simulink model "Controller"  (R2026a)
settings: Solver=FixedStepAuto  StopTime=inf  FixedStep=ControllerStepSize  MaxStep=Ts
PreLoadFcn:
  | % Position and velocity selectors from track state
  | % The filter initialization function used in this example is initcvekf that
  | % defines a state that is: [x;vx;y;vy;z;vz].
  | trackPosSelector = [1,0,0,0,0,0; 0,0,1,0,0,0];
  | assignin('base','trackPosSelector',trackPosSelector);
  | 
  | % Width of the ego path for MIO consideration(m)
  | assignin('base','egoPathWidth', single(3.5));
  | 
  | 
  | egoVehDyn.Mass = 1575;
  | egoVehDyn.CGToFrontAxle = 1.5149;
  | egoVehDyn.CGToRearAxle = 1.3042;
  | egoVehDyn.Cf = 19000;
  | assignin('base','egoVehDyn', egoVehDyn);
  | 
  | 
  | maxSteer = 1.13; % Maximum steering angle (rad)
  | assignin('base', 'maxSteer', maxSteer);
undefined symbols (not defined in the file or in its folder): accGapGain, accKi, accKp, accLaneWidth, accMaxAcceleration, accMinAcceleration, accStandstillGap, accTimeHeadway, AEB, ControllerStepSize, egoPathWidth, FCW, LaneWidth, Left, maxDecel, predictionHorizon, Right, Ts
libraries: simulink_extras x8, simulink x2, drivingvehiclecontroller x2, slpidlib x1, mpcadaslib x1
CloseFcn:
  | evalin('base','clear(''trackPosSelector'')');
  | evalin('base','clear(''egoPathWidth'')');
settings Model: Creator=The MathWorks, Inc.  LastModifiedBy=mraj
settings SolverCC: MinimalZcImpactIntegration=on
settings OptimizationCC: InlineInvariantSignals=on  InitFltsAndDblsToZero=on
settings HardwareCC: TargetLongLongMode=on
settings SFSimCC: SimTargetLang=C++
settings RTWCC: SystemTargetFile=ert.tlc  GenerateReport=on  BuildConfiguration=Faster Runs  IncludeHyperlinkInReport=on  LaunchReport=on  TargetLang=C++  GenerateTraceInfo=on  GenerateTraceReport=on  GenerateTraceReportSl=on  GenerateTraceReportSf=on  GenerateTraceReportEml=on  GenerateCodeMetricsReport=on  LargeConstantGeneration=WriteOnlyDNNConstantsToDataFiles  Description=Embedded Coder
settings CodeAppCC: MaxIdLength=63.0  CustomSymbolStrFcn=$N$M$F
settings ERTTargetCC: RootIOFormat=Structure reference  RTWCAPISignals=on  DynamicArrayContainerType=coder::array  TargetLangStandard=C++03 (ISO)  GenerateSampleERTMain=on  CombineSignalStateStructs=on  SuppressErrorStatus=on  CodeInterfacePackaging=C++ class  SupportVariableSizeSignals=on

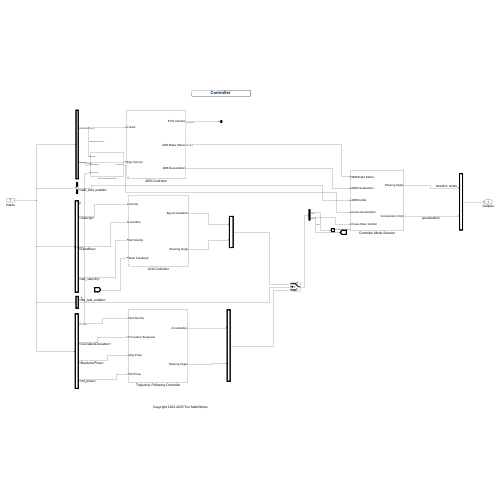
[thumbnail: Simulink's stored preview of the top-level diagram]
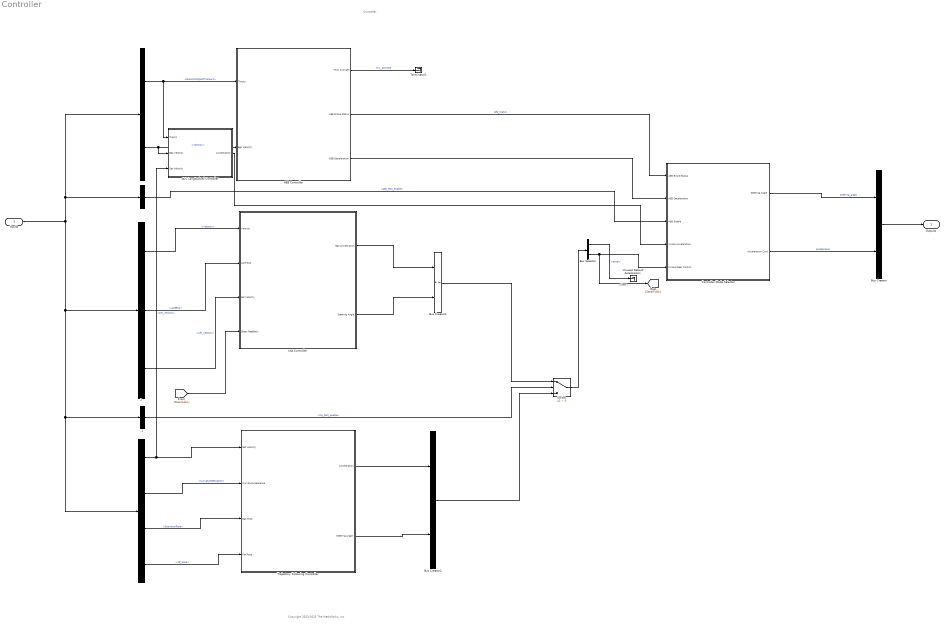
== system Controller ==
  note: Controller
  note: Copyright 2023-2025 The MathWorks, Inc.
  Inputs : Inport  OutDataTypeStr=Bus: BusController  BusOutputAsStruct=on
  "  " : BusSelector  OutputSignals=BusMultiObjectTracker1,BusActorPose.Velocity
  "    " : BusSelector  OutputSignals=set_velocity,BusRefPathInfo.BusDeviations.CurvatureDeviation,BusActorPose,BusRefPathInfo.ref_pose
  "     " : BusSelector  OutputSignals=aeb_test_enable
  "     1" : BusSelector  OutputSignals=lka_test_enable
  "    2" : BusSelector  OutputSignals=BusActorPose.Velocity,LaneBus,set_velocity
  ACC Longitudinal Controller : Subsystem
  AEB Controller : Subsystem  Variant=on  EmptyChoice=on
  Bus Creator : BusCreator  Inputs=2
  Bus Creator1 : BusCreator  Inputs=2  OutDataTypeStr=Bus: AccelSteerBus
      settings: InheritFromInputs=off
  Bus Creator2 : BusCreator  Inputs=2  OutDataTypeStr=Bus: AccelSteerBus
      settings: InheritFromInputs=off
  Bus Selector : BusSelector  OutputSignals=accel,steer
  Controller Mode Selector : Subsystem
  LKA Controller : Subsystem  Variant=on  EmptyChoice=on
  Switch : Switch  Criteria=u2 > Threshold  SaturateOnIntegerOverflow=off  InputSameDT=off  OutDataTypeStr=Inherit: Same as first input
  Terminator1 : Terminator
  Trajectory Following Controller : Subsystem
  Unused Default Acceleration : Terminator
  Outputs : Outport  OutDataTypeStr=Bus: BusVehicleCommands
  wires:
  "     "/1 -> Controller Mode Selector/3(AEB Enable)  "<aeb_test_enable>"
  Bus Creator/1 -> Outputs/1
  "    "/4 -> Trajectory Following Controller/4(Ref Pose)  "<ref_pose>"
  Controller Mode Selector/1(Steering Angle) -> Bus Creator/1  "steering_angle"
  "    "/2 -> Trajectory Following Controller/2(Curvature Sequence)  "<CurvatureDeviation>"
  "    "/3 -> Trajectory Following Controller/3(Ego Pose)  "<BusActorPose>"
  Controller Mode Selector/2(Acceleration Cmd) -> Bus Creator/2  "acceleration"
  Switch/1 -> Bus Selector/1
  Inputs/1 -> "  "/1, "     "/1, "    2"/1, "     1"/1, "    "/1
  "    2"/1 -> LKA Controller/1(Velocity)  "<Velocity>"
  LKA Controller/1(Ego Acceleration) -> Bus Creator1/1
  "    2"/3 -> LKA Controller/3(Set Velocity)  "<set_velocity>"
  "    2"/2 -> LKA Controller/2(Lane Bus)  "<LaneBus>"
  LKA Controller/2(Steering Angle) -> Bus Creator1/2
  Bus Creator1/1 -> Switch/1
  "     1"/1 -> Switch/2  "<lka_test_enable>"
  Bus Creator2/1 -> Switch/3
  Trajectory Following Controller/1(Acceleration) -> Bus Creator2/1
  Trajectory Following Controller/2(Steering Angle) -> Bus Creator2/2
  [SteerFdbk] -> LKA Controller/4(Steer Feedback)
  AEB Controller/1(FCW Activate) -> Terminator1/1  "fcw_activate"
  AEB Controller/2(AEB Brake Status) -> Controller Mode Selector/1(AEB Brake Status)  "aeb_status"
  AEB Controller/3(AEB Deceleration) -> Controller Mode Selector/2(AEB Deceleration)
  Bus Selector/1 -> Unused Default Acceleration/1  "<accel>"
  ACC Longitudinal Controller/1(Acceleration) -> Controller Mode Selector/4(Cruise Acceleration)
  "  "/2 -> ACC Longitudinal Controller/2(Ego Velocity), AEB Controller/2(Ego Velocity)  "<Velocity>"
  "  "/1 -> ACC Longitudinal Controller/1(Tracks), AEB Controller/1(Tracks)  "<BusMultiObjectTracker1>"
  Bus Selector/2 -> [SteerFdbk], Controller Mode Selector/5(Cruise Steer Control)  "<steer>"
  "    "/1 -> ACC Longitudinal Controller/3(Set Velocity), Trajectory Following Controller/1(Set Velocity)  "<set_velocity>"

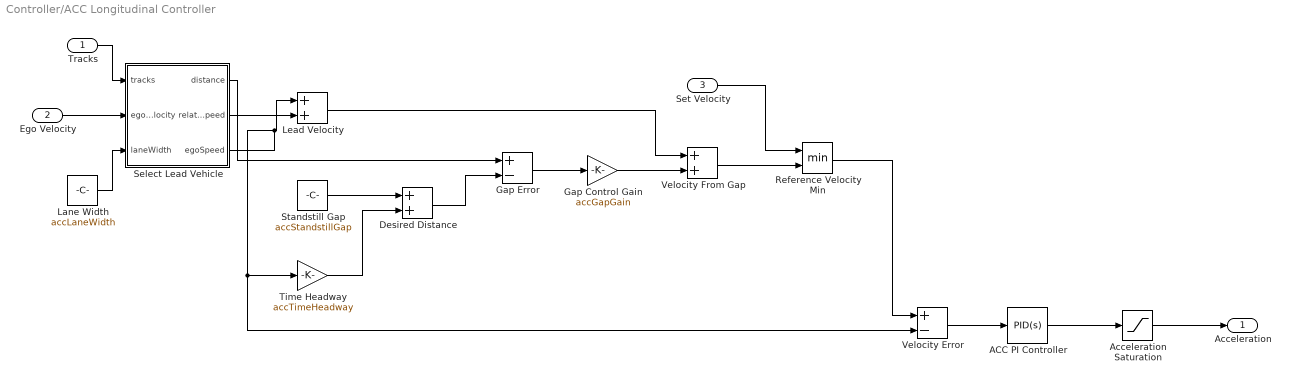
== system Controller/ACC Longitudinal Controller ==
  Tracks : Inport
  Ego Velocity : Inport  Port=2
  Set Velocity : Inport  Port=3
  ACC PI Controller : slpidlib/PID Controller  Controller=PID  Form=Parallel  TimeDomain=Continuous-time  UseExternalTs=off  SampleTime=-1  IntegratorMethod=Forward Euler  FilterMethod=Forward Euler  ControllerParametersSource=internal  P=accKp  I=accKi  UseKiTs=off  D=0  UseExternalDerivativeSource=off  N=100  UseFilter=on  TunerSelectOption=Transfer Function Based (PID Tuner App)  InitialConditionSource=internal  InitialConditionForIntegrator=0  InitialConditionForFilter=0  DifferentiatorICPrevScaledInput=0  ExternalReset=none  TrackingMode=off  Kt=1  LimitOutput=off  SatLimitsSource=internal  UpperSaturationLimit=inf  LowerSaturationLimit=-inf  LinearizeAsGain=on  AntiWindupMode=none  Kb=1  LimitIntegrator=off  UpperIntegratorSaturationLimit=inf  LowerIntegratorSaturationLimit=-inf  POutMin=[]  POutMax=[]  IOutMin=[]  IOutMax=[]  DOutMin=[]  DOutMax=[]  NOutMin=[]  NOutMax=[]  SumOutMin=[]  SumOutMax=[]  SaturationOutMin=[]  SaturationOutMax=[]  PParamMin=[]  PParamMax=[]  IParamMin=[]  IParamMax=[]  DParamMin=[]  DParamMax=[]  NParamMin=[]  NParamMax=[]  KbParamMin=[]  KbParamMax=[]  KtParamMin=[]  KtParamMax=[]  KbOutMin=[]  KbOutMax=[]  KtOutMin=[]  KtOutMax=[]  IntegratorOutMin=[]  IntegratorOutMax=[]  FilterOutMin=[]  FilterOutMax=[]  SumI1OutMin=[]  SumI1OutMax=[]  SumI2OutMin=[]  SumI2OutMax=[]  SumI3OutMin=[]  SumI3OutMax=[]  SumI4OutMin=[]  SumI4OutMax=[]  SumDOutMin=[]  SumDOutMax=[]  DifferentiatorOutMin=[]  DifferentiatorOutMax=[]  FilterDiffOutCoefMin=[]  FilterDiffOutCoefMax=[]  ReciprocalOutMin=[]  ReciprocalOutMax=[]  SumDenOutMin=[]  SumDenOutMax=[]  SumNumOutMin=[]  SumNumOutMax=[]  DivideOutMin=[]  DivideOutMax=[]  UdiffTsProdOutMin=[]  UdiffTsProdOutMax=[]  NTsProdOutMin=[]  NTsProdOutMax=[]  UintegralTsProdOutMin=[]  UintegralTsProdOutMax=[]  UngainTsProdOutMin=[]  UngainTsProdOutMax=[]  ClampingZeroOutDataTypeStr=Inherit: Inherit via back propagation  ClampingZeroOutMin=[]  ClampingZeroOutMax=[]  FilterDenConstantOutDataTypeStr=Inherit: Inherit via back propagation  FilterDenConstantOutMin=[]  FilterDenConstantOutMax=[]  PCopyOutDataTypeStr=Inherit: Inherit via back propagation  PCopyOutMin=[]  PCopyOutMax=[]  NCopyOutDataTypeStr=Inherit: Inherit via back propagation  NCopyOutMin=[]  NCopyOutMax=[]  IntegratorContinuousStateAttributes=''  IntegratorStateMustResolveToSignalObject=off  IntegratorRTWStateStorageClass=Auto  FilterContinuousStateAttributes=''  FilterStateMustResolveToSignalObject=off  FilterRTWStateStorageClass=Auto  ParallelPVariant=InternalParameters  IdealPVariant=Disabled  IVariant=InternalParameters  DVariant=InternalParameters  IntegratorVariant=Continuous  SatVariant=Disabled  AWVariant=Passthrough  PCopyVariant=Disabled  TRVariant=Disabled  FdbkBlocksVariant=Forward  IdealPFdbkVariant=Disabled  SatFdbkVariant=Disabled  DerivativeFilterVariant=ContFilter  NVariant=InternalParameters  NCopyVariant=Disabled  FilterICVariant=InternalICsFilter  IntegratorICVariant=InternalICs  ExternalResetVariant=Disabled  TRSumVariant=Passthrough  SumFdbkVariant=Disabled  SumVariant=Sum_PID  TsampFilterVariant=InternalTs  TsampNgainVariant=Passthrough  TsampIntegralVariant=Disabled_SignalSpec  ExternalSaturationOutDataTypeStr=Inherit: Same as second input  DerivativeSourceVariant=ErrorSignal  PreIntVariant=InternalPreInt
  Acceleration Saturation : Saturate  UpperLimit=accMaxAcceleration  LowerLimit=accMinAcceleration
  Desired Distance : Sum
  Gap Control Gain : Gain  Gain=accGapGain
  Gap Error : Sum  Inputs=+-
  Lane Width : Constant  Value=accLaneWidth
  Lead Velocity : Sum
  Reference Velocity Min : MinMax  Inputs=2
  Select Lead Vehicle : MATLAB Function  TreatAsAtomicUnit=on
  Standstill Gap : Constant  Value=accStandstillGap
  Time Headway : Gain  Gain=accTimeHeadway
  Velocity Error : Sum  Inputs=+-
  Velocity From Gap : Sum
  Acceleration : Outport
  wires:
  Select Lead Vehicle/2(relativeSpeed) -> Lead Velocity/2
  Select Lead Vehicle/3(egoSpeed) -> Time Headway/1, Velocity Error/2, Lead Velocity/1
  Lane Width/1 -> Select Lead Vehicle/3(laneWidth)
  Ego Velocity/1 -> Select Lead Vehicle/2(egoVelocity)
  Tracks/1 -> Select Lead Vehicle/1(tracks)
  Standstill Gap/1 -> Desired Distance/1
  Time Headway/1 -> Desired Distance/2
  Select Lead Vehicle/1(distance) -> Gap Error/1
  Desired Distance/1 -> Gap Error/2
  Gap Error/1 -> Gap Control Gain/1
  Lead Velocity/1 -> Velocity From Gap/1
  Gap Control Gain/1 -> Velocity From Gap/2
  Set Velocity/1 -> Reference Velocity Min/1
  Velocity From Gap/1 -> Reference Velocity Min/2
  Reference Velocity Min/1 -> Velocity Error/1
  Velocity Error/1 -> ACC PI Controller/1
  ACC PI Controller/1 -> Acceleration Saturation/1
  Acceleration Saturation/1 -> Acceleration/1

== system Controller/AEB Controller ==
  Tracks : Inport
  Ego Velocity : Inport  Port=2
  AEB Controller : Subsystem  VariantControl=aebEnable==1
  FCW Activate : Outport
  AEB Brake Status : Outport  Port=2
  AEB Deceleration : Outport  Port=3

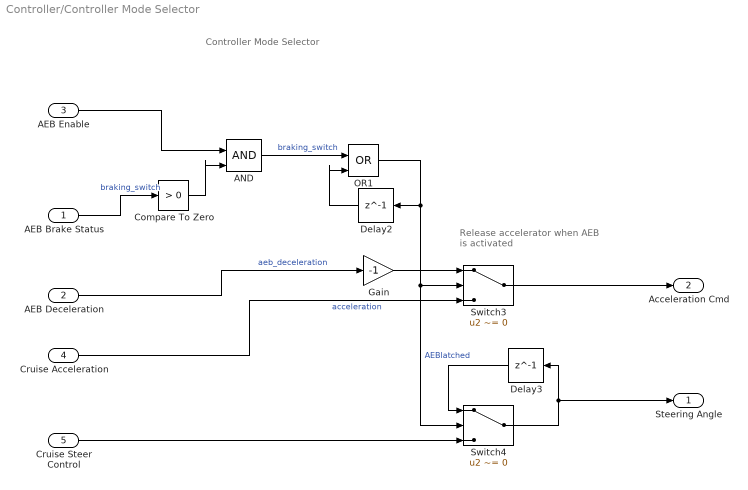
== system Controller/Controller Mode Selector ==
  note: Release accelerator when AEB is activated
  note: Controller Mode Selector
  AEB Brake Status : Inport
  AEB Deceleration : Inport  Port=2
  AEB Enable : Inport  Port=3
  Cruise Acceleration : Inport  Port=4
  Cruise Steer Control : Inport  Port=5
  AND : Logic  IconShape=distinctive  AllPortsSameDT=off  OutDataTypeStr=boolean
  Compare To Zero : simulink/Logic and Bit Operations/Compare To Zero  relop=>  OutDataTypeStr=boolean
  Delay2 : Delay  DelayLength=1
  Delay3 : Delay  DelayLength=1
  Gain : Gain  Gain=-1
  OR1 : Logic  Operator=OR  IconShape=distinctive  AllPortsSameDT=off  OutDataTypeStr=boolean
  Switch3 : Switch  Criteria=u2 ~= 0  SaturateOnIntegerOverflow=off  InputSameDT=off
  Switch4 : Switch  Criteria=u2 ~= 0  SaturateOnIntegerOverflow=off  InputSameDT=off
  Steering Angle : Outport
  Acceleration Cmd : Outport  Port=2
  wires:
  AND/1 -> OR1/1  "braking_switch"
  AEB Deceleration/1 -> Gain/1  "aeb_deceleration"
  Switch3/1 -> Acceleration Cmd/1
  Delay2/1 -> OR1/2
  Switch4/1 -> Steering Angle/1, Delay3/1
  Cruise Steer Control/1 -> Switch4/3
  Delay3/1 -> Switch4/1
  Gain/1 -> Switch3/1
  OR1/1 -> Delay2/1, Switch4/2, Switch3/2  "AEBlatched"
  Cruise Acceleration/1 -> Switch3/3  "acceleration"
  AEB Brake Status/1 -> Compare To Zero/1  "braking_switch"
  AEB Enable/1 -> AND/1
  Compare To Zero/1 -> AND/2

== system Controller/LKA Controller ==
  Velocity : Inport
  Lane Bus : Inport  Port=2
  Set Velocity : Inport  Port=3
  Steer Feedback : Inport  Port=4
  LKA Controller : Subsystem  VariantControl=lkaEnable==1
  Ego Acceleration : Outport
  Steering Angle : Outport  Port=2

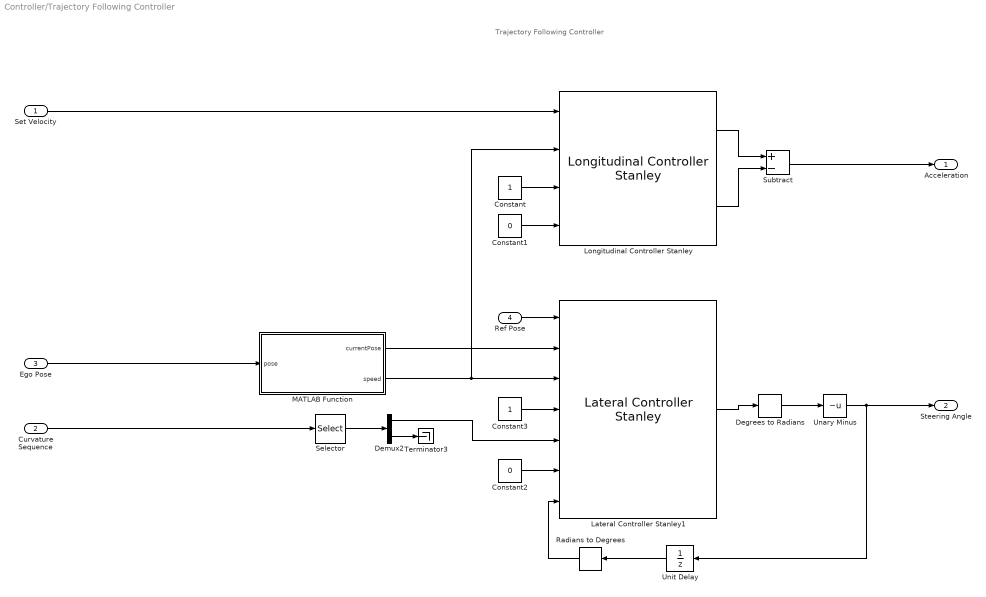
== system Controller/Trajectory Following Controller ==
  note: Trajectory Following Controller
  Set Velocity : Inport  SampleTime=ControllerStepSize
  Curvature Sequence : Inport  Port=2  SampleTime=ControllerStepSize
  Ego Pose : Inport  Port=3  SampleTime=ControllerStepSize
  Ref Pose : Inport  Port=4
  Constant : Constant  SampleTime=ControllerStepSize
  Constant1 : Constant  Value=0
  Constant2 : Constant  Value=0
  Constant3 : Constant  SampleTime=ControllerStepSize
  Degrees to Radians : simulink_extras/Transformations/Degrees to Radians
  Demux2 : Demux  Outputs=2
  Lateral Controller Stanley1 : drivingvehiclecontroller/Lateral Controller Stanley  ModelType=Dynamic bicycle model  PositionGainF=5  PositionGainR=2.5  YawRateGain=0.2  DelayGain=0.5  VehicleMass=egoVehDyn.Mass  Lf=egoVehDyn.CGToFrontAxle  Lr=egoVehDyn.CGToRearAxle  TireStiffness=egoVehDyn.Cf  Wheelbase=2.8  MaxSteeringAngle=rad2deg(maxSteer)
  Longitudinal Controller Stanley : drivingvehiclecontroller/Longitudinal Controller Stanley  Kp=2.5  Ki=1  SampleTime=ControllerStepSize  MaxAcceleration=maxAcc  MaxDeceleration=-maxDecel
  MATLAB Function : MATLAB Function  TreatAsAtomicUnit=on
  Radians to Degrees : simulink_extras/Transformations/Radians to Degrees
  Selector : Selector  InputPortWidth=predictionHorizon  IndexOptions=Index vector (dialog)  Indices=[1 3]  OutputSizes=1
  Subtract : Sum  Inputs=+-
  Terminator3 : Terminator
  Unary Minus : UnaryMinus
  Unit Delay : UnitDelay  SampleTime=-1
  Acceleration : Outport
  Steering Angle : Outport  Port=2
  wires:
  Curvature Sequence/1 -> Selector/1
  Subtract/1 -> Acceleration/1
  Unary Minus/1 -> Steering Angle/1, Unit Delay/1
  Degrees to Radians/1 -> Unary Minus/1
  Lateral Controller Stanley1/1 -> Degrees to Radians/1
  Ref Pose/1 -> Lateral Controller Stanley1/1
  Constant2/1 -> Lateral Controller Stanley1/6
  Radians to Degrees/1 -> Lateral Controller Stanley1/7
  Unit Delay/1 -> Radians to Degrees/1
  Selector/1 -> Demux2/1
  Demux2/2 -> Terminator3/1
  Demux2/1 -> Lateral Controller Stanley1/5
  Constant/1 -> Longitudinal Controller Stanley/3
  Constant1/1 -> Longitudinal Controller Stanley/4
  Longitudinal Controller Stanley/2 -> Subtract/2
  Longitudinal Controller Stanley/1 -> Subtract/1
  MATLAB Function/2(speed) -> Longitudinal Controller Stanley/2, Lateral Controller Stanley1/3
  Set Velocity/1 -> Longitudinal Controller Stanley/1
  Constant3/1 -> Lateral Controller Stanley1/4
  MATLAB Function/1(currentPose) -> Lateral Controller Stanley1/2
  Ego Pose/1 -> MATLAB Function/1(pose)

== system Controller/AEB Controller/AEB Controller ==
  note: AEB Controller
  Tracks : Inport  OutDataTypeStr=Bus: BusMultiObjectTracker1  SampleTime=ControllerStepSize  BusOutputAsStruct=on
  Ego Velocity : Inport  Port=2  PortDimensions=[1 3]
  Constant : Constant  Value=egoPathWidth
  Ego Speed : MATLAB Function  TreatAsAtomicUnit=on
  Emergency Braking Controller : Subsystem
  Find MIO : MATLAB Function  TreatAsAtomicUnit=on
  Position Selector : Constant  Value=trackPosSelector
  Terminator : Terminator
  FCW Activate : Outport  OutDataTypeStr=uint8  PortDimensions=1  VectorParamsAs1DForOutWhenUnconnected=off
  AEB Brake Status : Outport  Port=2  OutDataTypeStr=uint8  PortDimensions=1  VectorParamsAs1DForOutWhenUnconnected=off
  AEB Deceleration : Outport  Port=3
  wires:
  Find MIO/2(vx) -> Emergency Braking Controller/2(MIO Velocity)
  Position Selector/1 -> Find MIO/2(positionSelector)
  Ego Velocity/1 -> Ego Speed/1(velocity)
  Emergency Braking Controller/1(FCW Activate) -> FCW Activate/1  "fcw_activate"
  Emergency Braking Controller/3(Deceleration) -> AEB Deceleration/1
  Ego Speed/1(speed) -> Find MIO/4(egoSpeed), Emergency Braking Controller/4(Longitudinal Velocity)  "ego_velocity"
  Find MIO/1(x) -> Emergency Braking Controller/1(MIO Distance)
  Constant/1 -> Find MIO/3(laneWidth)
  Emergency Braking Controller/2(AEB Status) -> AEB Brake Status/1  "aeb_status"
  Find MIO/3(mioTrack) -> Terminator/1
  Find MIO/4(relativeYawAngle) -> Emergency Braking Controller/3(relativeYawAngle)
  Tracks/1 -> Find MIO/1(confirmedTracks)

== system Controller/LKA Controller/LKA Controller ==
  Velocity : Inport
  Lane Bus : Inport  Port=2
  Set Velocity : Inport  Port=3
  Steer Feedback : Inport  Port=4
  Ego Speed : MATLAB Function  TreatAsAtomicUnit=on
  EstimateLaneCenter : Subsystem  TreatAsAtomicUnit=on  VariantControl=v2
      settings: RTWFileNameOpts=Use function name
  Lane Following Controller : Subsystem
  Pack Lane Detections : Subsystem
  Preview Curvature : Subsystem  VariantControl=v2
      settings: RTWFileNameOpts=Use function name
  Ego Acceleration : Outport
  Steering Angle : Outport  Port=2
  wires:
  Preview Curvature/3(Relative Yaw Angle) -> Lane Following Controller/4(relative_yaw_angle)
  Ego Speed/1(speed) -> Preview Curvature/1(Longitudinal Velocity), Lane Following Controller/1(Ego Speed)  "ego_velocity"
  Velocity/1 -> Ego Speed/1(velocity)
  EstimateLaneCenter/1(LaneCenter) -> Preview Curvature/2(Lane Center)
  Preview Curvature/1(Previewed Curvature) -> Lane Following Controller/2(Previewed Curvature)
  Lane Following Controller/2(steerCMD) -> Steering Angle/1  "steering_angle"
  Set Velocity/1 -> Lane Following Controller/5(set_velocity)
  Pack Lane Detections/1(LanesOut) -> EstimateLaneCenter/1(LaneDetections)  "lane_detections"
  Preview Curvature/2(Lateral Deviation) -> Lane Following Controller/3(lateral_deviation)
  Steer Feedback/1 -> Lane Following Controller/6(Steering Angle)
  Lane Following Controller/1(accelCMD) -> Ego Acceleration/1  "ego_acceleration"
  Lane Bus/1 -> Pack Lane Detections/1(LanesIn)

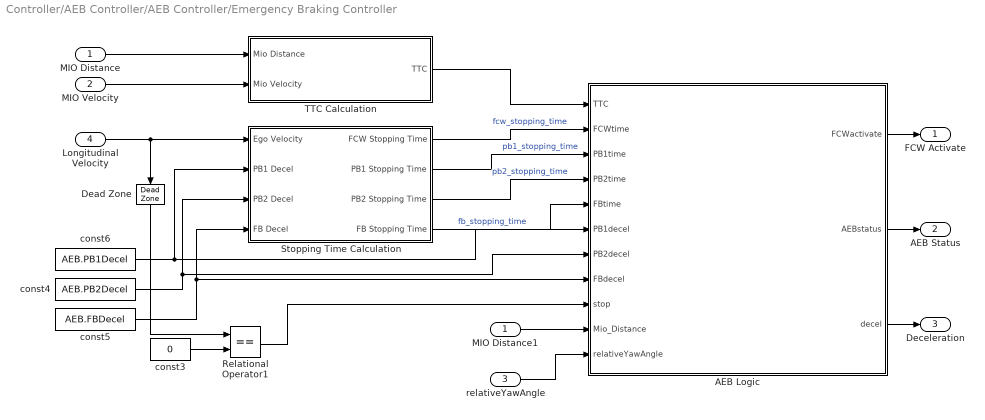
== system Controller/AEB Controller/AEB Controller/Emergency Braking Controller ==
  MIO Distance : Inport
  MIO Velocity : Inport  Port=2
  relativeYawAngle : Inport  Port=3
  Longitudinal Velocity : Inport  Port=4
  AEB Logic : Stateflow chart  TreatAsAtomicUnit=on
  Dead Zone : DeadZone  LowerValue=-inf  UpperValue=0.001
  MIO Distance1 : InportShadow
  Relational Operator1 : RelationalOperator  Operator===  OutDataTypeStr=boolean  RndMeth=Simplest  InputSameDT=off
  Stopping Time Calculation : Subsystem
  TTC Calculation : Subsystem
  const3 : Constant  Value=0  SampleTime=-1
  const4 : Constant  Value=AEB.PB2Decel  SampleTime=-1
  const5 : Constant  Value=AEB.FBDecel  SampleTime=-1
  const6 : Constant  Value=AEB.PB1Decel  SampleTime=-1
  FCW Activate : Outport  VectorParamsAs1DForOutWhenUnconnected=off
  AEB Status : Outport  Port=2  VectorParamsAs1DForOutWhenUnconnected=off
  Deceleration : Outport  Port=3  OutDataTypeStr=double  VectorParamsAs1DForOutWhenUnconnected=off
  wires:
  AEB Logic/3(decel) -> Deceleration/1
  const4/1 -> AEB Logic/7(PB2decel), Stopping Time Calculation/3(PB2 Decel)
  const5/1 -> Stopping Time Calculation/4(FB Decel), AEB Logic/8(FBdecel)
  AEB Logic/2(AEBstatus) -> AEB Status/1
  const3/1 -> Relational Operator1/2
  const6/1 -> AEB Logic/6(PB1decel), Stopping Time Calculation/2(PB1 Decel)
  Stopping Time Calculation/3(PB2 Stopping Time) -> AEB Logic/4(PB2time)  "pb2_stopping_time"
  Stopping Time Calculation/2(PB1 Stopping Time) -> AEB Logic/3(PB1time)  "pb1_stopping_time"
  Stopping Time Calculation/4(FB Stopping Time) -> AEB Logic/5(FBtime)  "fb_stopping_time"
  Stopping Time Calculation/1(FCW Stopping Time) -> AEB Logic/2(FCWtime)  "fcw_stopping_time"
  AEB Logic/1(FCWactivate) -> FCW Activate/1
  MIO Distance/1 -> TTC Calculation/1(Mio Distance)
  MIO Velocity/1 -> TTC Calculation/2(Mio Velocity)
  TTC Calculation/1(TTC) -> AEB Logic/1(TTC)
  Longitudinal Velocity/1 -> Dead Zone/1, Stopping Time Calculation/1(Ego Velocity)
  Relational Operator1/1 -> AEB Logic/9(stop)
  MIO Distance1/1 -> AEB Logic/10(Mio_Distance)
  relativeYawAngle/1 -> AEB Logic/11(relativeYawAngle)
  Dead Zone/1 -> Relational Operator1/1

== system Controller/LKA Controller/LKA Controller/EstimateLaneCenter ==
  note: Input: LaneDetections
      | Description: Computes centerline from detected lane boundaries
      | Output: LaneCenter
  LaneDetections : Inport
  CenterFromLeft : Subsystem  TreatAsAtomicUnit=on
  CenterFromLeftAndRight : Subsystem  TreatAsAtomicUnit=on
  CenterFromNone : Subsystem  TreatAsAtomicUnit=on
  CenterFromRight : Subsystem  TreatAsAtomicUnit=on
  Lane Detections1 : InportShadow
  Lane Detections2 : InportShadow
  Lane Detections3 : InportShadow
  MATLAB Function : MATLAB Function  TreatAsAtomicUnit=on
  Merge : Merge  Inputs=4
  LaneCenter : Outport
  wires:
  CenterFromRight/1(Center) -> Merge/3
  Lane Detections2/1 -> CenterFromLeft/1(Lanes)
  Lane Detections3/1 -> CenterFromRight/1(Lanes)
  MATLAB Function/2(centerFromLeftFunction()) -> CenterFromLeft/Trigger
  CenterFromNone/1(NewCenter) -> Merge/4
  MATLAB Function/1(centerFromLeftAndRightFunction()) -> CenterFromLeftAndRight/Trigger
  Merge/1 -> CenterFromNone/1(OldCenter), LaneCenter/1
  CenterFromLeftAndRight/1(Center) -> Merge/1
  LaneDetections/1 -> MATLAB Function/1(lanes)
  Lane Detections1/1 -> CenterFromLeftAndRight/1(Lanes)
  MATLAB Function/3(centerFromRigthFunction()) -> CenterFromRight/Trigger
  MATLAB Function/4(centerFromNoneFunction()) -> CenterFromNone/Trigger
  CenterFromLeft/1(Center) -> Merge/2

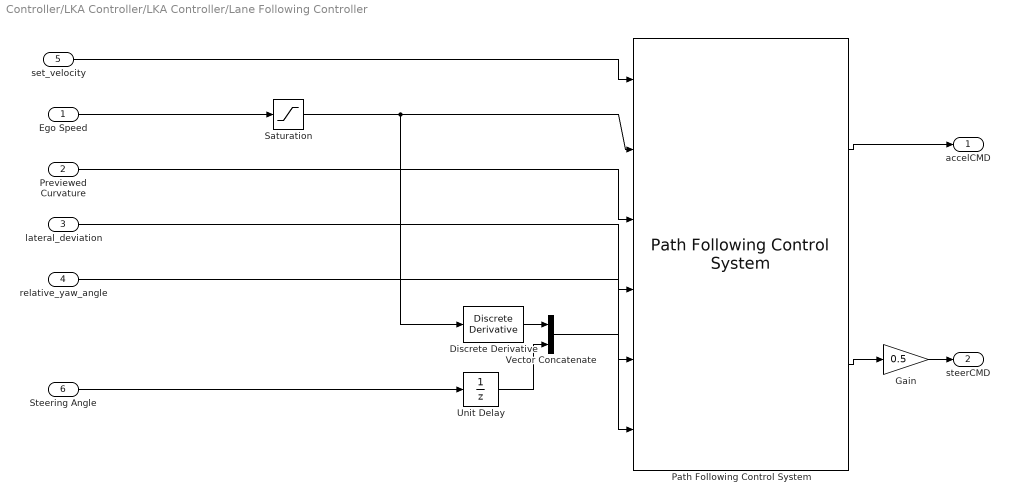
== system Controller/LKA Controller/LKA Controller/Lane Following Controller ==
  Ego Speed : Inport
  Previewed Curvature : Inport  Port=2
  lateral_deviation : Inport  Port=3
  relative_yaw_angle : Inport  Port=4
  set_velocity : Inport  Port=5
  Steering Angle : Inport  Port=6
  Discrete Derivative : simulink/Discrete/Discrete Derivative  gainval=1.0  ICPrevScaledInput=0.0  OutMin=[]  OutMax=[]  OutDataType=fixdt(1, 16)  OutScaling=2^-10  DoSatur=off
  Gain : Gain  Gain=0.5
  Path Following Control System : mpcadaslib/Path Following Control System  VariantControl=Variant2  ModelType=Use vehicle parameters  VehicleMass=egoVehDyn.Mass  VehicleYawInertia=egoVehDyn.YawMomentOfInertia  LengthToFront=egoVehDyn.CGToFrontAxle  LengthToRear=egoVehDyn.CGToRearAxle  FrontTireStiffness=egoVehDyn.Cf  RearTireStiffness=egoVehDyn.Cr  AccelTimeConstant=Ts  EgoModelMatrixA=[-2,zeros(1,3);1,zeros(1,3);zeros(1,2),-4.4021,-12.4603;zeros(1,2),1.3913,-5.1868]  EgoModelMatrixB=[2,zeros(1,3);zeros(1,2),24.1270,15.8609]'  EgoModelMatrixC=[zeros(3,1),eye(3)]  InitialLongVel=egoVehDyn.VLong0  TransportLag=0  spaceCtrl=off  DefaultSpacing=12  MinSteering=minSteer  umin_ext=off  MaxSteering=maxSteer  umax_ext=off  MinAcceleration=minAcc  amin_ext=off  MaxAcceleration=maxAcc  amax_ext=off  Ts=Ts*7  PredictionHorizon=10  ControlHorizon=2  LongWeight=0.01  LateralWeight=20  AccelRateWeight=0.01  SteerRateWeight=20  suboptimal=on  maxiter=100  datatypeopt=double  optmode=off  trackmode=on
  Saturation : Saturate  UpperLimit=100  LowerLimit=0.00001
  Unit Delay : UnitDelay  SampleTime=Ts
  Vector Concatenate : Concatenate
  accelCMD : Outport
  steerCMD : Outport  Port=2
  wires:
  Path Following Control System/1 -> accelCMD/1
  Ego Speed/1 -> Saturation/1
  set_velocity/1 -> Path Following Control System/1
  Saturation/1 -> Discrete Derivative/1, Path Following Control System/2
  relative_yaw_angle/1 -> Path Following Control System/5
  lateral_deviation/1 -> Path Following Control System/4
  Path Following Control System/2 -> Gain/1
  Vector Concatenate/1 -> Path Following Control System/6
  Discrete Derivative/1 -> Vector Concatenate/1
  Steering Angle/1 -> Unit Delay/1
  Unit Delay/1 -> Vector Concatenate/2
  Previewed Curvature/1 -> Path Following Control System/3
  Gain/1 -> steerCMD/1

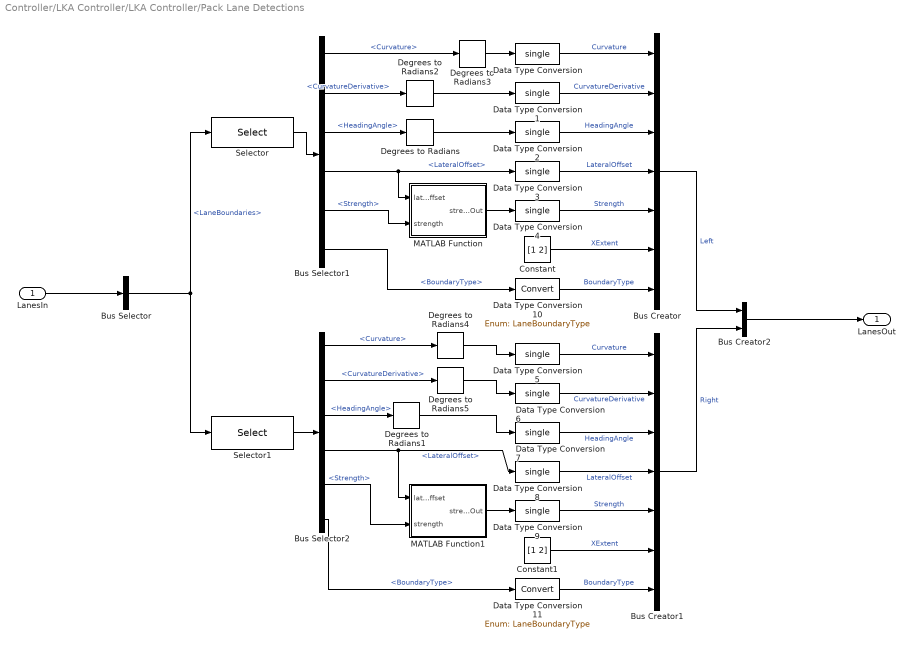
== system Controller/LKA Controller/LKA Controller/Pack Lane Detections ==
  LanesIn : Inport
  Bus Creator : BusCreator  Inputs=7  OutDataTypeStr=Bus: LaneSensorBoundaries
  Bus Creator1 : BusCreator  Inputs=7  OutDataTypeStr=Bus: LaneSensorBoundaries
  Bus Creator2 : BusCreator  Inputs=Left,Right  OutDataTypeStr=Bus: LaneSensor
  Bus Selector : BusSelector  OutputSignals=LaneBoundaries
  Bus Selector1 : BusSelector  OutputSignals=Curvature,CurvatureDerivative,HeadingAngle,LateralOffset,Strength,BoundaryType
  Bus Selector2 : BusSelector  OutputSignals=Curvature,CurvatureDerivative,HeadingAngle,LateralOffset,Strength,BoundaryType
  Constant : Constant  Value=[1 2]  OutDataTypeStr=single
  Constant1 : Constant  Value=[1 2]  OutDataTypeStr=single
  Data Type Conversion{,1..9} (10 alike) : DataTypeConversion  OutDataTypeStr=single  SaturateOnIntegerOverflow=off  RndMeth=Floor
  Data Type Conversion10 : DataTypeConversion  OutDataTypeStr=Enum: LaneBoundaryType  SaturateOnIntegerOverflow=off  RndMeth=Floor
  Data Type Conversion11 : DataTypeConversion  OutDataTypeStr=Enum: LaneBoundaryType  SaturateOnIntegerOverflow=off  RndMeth=Floor
  Degrees to Radians{,1..5} (6 alike) : simulink_extras/Transformations/Degrees to Radians
  MATLAB Function : MATLAB Function  TreatAsAtomicUnit=on
  MATLAB Function1 : MATLAB Function  TreatAsAtomicUnit=on
  Selector : Selector  InputPortWidth=2  IndexOptions=Index vector (dialog)  Indices=1  OutputSizes=1  RuntimeRangeChecks=on
  Selector1 : Selector  InputPortWidth=2  IndexOptions=Index vector (dialog)  Indices=2  OutputSizes=1
  LanesOut : Outport  VectorParamsAs1DForOutWhenUnconnected=off
  wires:
  LanesIn/1 -> Bus Selector/1
  Bus Selector/1 -> Selector/1, Selector1/1  "<LaneBoundaries>"
  Selector/1 -> Bus Selector1/1
  Bus Selector1/2 -> Degrees to Radians2/1  "<CurvatureDerivative>"
  Bus Selector1/1 -> Degrees to Radians3/1  "<Curvature>"
  Bus Selector1/3 -> Degrees to Radians/1  "<HeadingAngle>"
  Bus Selector1/4 -> Data Type Conversion3/1, MATLAB Function/1(laterOffset)  "<LateralOffset>"
  Data Type Conversion/1 -> Bus Creator/1  "Curvature"
  Data Type Conversion1/1 -> Bus Creator/2  "CurvatureDerivative"
  Data Type Conversion2/1 -> Bus Creator/3  "HeadingAngle"
  Data Type Conversion3/1 -> Bus Creator/4  "LateralOffset"
  Data Type Conversion4/1 -> Bus Creator/5  "Strength"
  Data Type Conversion9/1 -> Bus Creator1/5  "Strength"
  Data Type Conversion6/1 -> Bus Creator1/2  "CurvatureDerivative"
  Data Type Conversion7/1 -> Bus Creator1/3  "HeadingAngle"
  Data Type Conversion8/1 -> Bus Creator1/4  "LateralOffset"
  Data Type Conversion5/1 -> Bus Creator1/1  "Curvature"
  Bus Selector2/1 -> Degrees to Radians4/1  "<Curvature>"
  Selector1/1 -> Bus Selector2/1
  Bus Selector2/4 -> MATLAB Function1/1(laterOffset), Data Type Conversion8/1  "<LateralOffset>"
  Bus Selector2/2 -> Degrees to Radians5/1  "<CurvatureDerivative>"
  Bus Selector2/3 -> Degrees to Radians1/1  "<HeadingAngle>"
  Bus Creator2/1 -> LanesOut/1
  Bus Creator/1 -> Bus Creator2/1  "Left"
  Bus Creator1/1 -> Bus Creator2/2  "Right"
  Constant/1 -> Bus Creator/6  "XExtent"
  Bus Selector1/6 -> Data Type Conversion10/1  "<BoundaryType>"
  Bus Selector2/6 -> Data Type Conversion11/1  "<BoundaryType>"
  Constant1/1 -> Bus Creator1/6  "XExtent"
  Data Type Conversion10/1 -> Bus Creator/7  "BoundaryType"
  Data Type Conversion11/1 -> Bus Creator1/7  "BoundaryType"
  MATLAB Function/1(strengthOut) -> Data Type Conversion4/1
  Bus Selector1/5 -> MATLAB Function/2(strength)  "<Strength>"
  MATLAB Function1/1(strengthOut) -> Data Type Conversion9/1
  Bus Selector2/5 -> MATLAB Function1/2(strength)  "<Strength>"
  Degrees to Radians1/1 -> Data Type Conversion7/1
  Degrees to Radians4/1 -> Data Type Conversion5/1
  Degrees to Radians5/1 -> Data Type Conversion6/1
  Degrees to Radians3/1 -> Data Type Conversion/1
  Degrees to Radians2/1 -> Data Type Conversion1/1
  Degrees to Radians/1 -> Data Type Conversion2/1

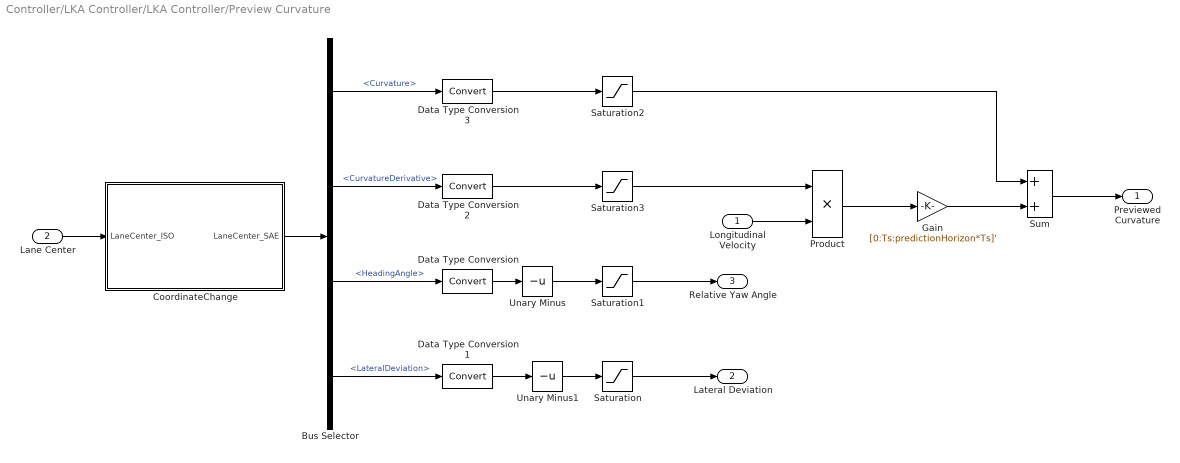
== system Controller/LKA Controller/LKA Controller/Preview Curvature ==
  Longitudinal Velocity : Inport
  Lane Center : Inport  Port=2
  Bus Selector : BusSelector  OutputSignals=Curvature,CurvatureDerivative,HeadingAngle,LateralDeviation
  CoordinateChange : Subsystem
  Data Type Conversion{,1..3} (4 alike) : DataTypeConversion  SaturateOnIntegerOverflow=off  RndMeth=Floor
  Gain : Gain  Gain=[0:Ts:predictionHorizon*Ts]'
      settings: AttributesFormatString=|
      | ----------------------------------------
      | Gain = %<Gain>
  Product : Product
  Saturation : Saturate
      settings: AttributesFormatString=|
      | -------------------------------
      | UpperLimit = %<UpperLimit>
      | LowerLimit = %<LowerLimit>
  Saturation1 : Saturate  UpperLimit=0.6  LowerLimit=-0.6
      settings: AttributesFormatString=|
      | -------------------------------
      | UpperLimit = %<UpperLimit>
      | LowerLimit = %<LowerLimit>
  Saturation2 : Saturate  UpperLimit=0.15  LowerLimit=-0.15
      settings: AttributesFormatString=|
      | -------------------------------
      | UpperLimit = %<UpperLimit>
      | LowerLimit = %<LowerLimit>
  Saturation3 : Saturate  UpperLimit=0.06  LowerLimit=-0.06
      settings: AttributesFormatString=|
      | -------------------------------
      | UpperLimit = %<UpperLimit>
      | LowerLimit = %<LowerLimit>
  Sum : Sum
  Unary Minus : UnaryMinus
  Unary Minus1 : UnaryMinus
  Previewed Curvature : Outport  VectorParamsAs1DForOutWhenUnconnected=off
  Lateral Deviation : Outport  Port=2  VectorParamsAs1DForOutWhenUnconnected=off
  Relative Yaw Angle : Outport  Port=3  VectorParamsAs1DForOutWhenUnconnected=off
  wires:
  Lane Center/1 -> CoordinateChange/1(LaneCenter_ISO)
  Bus Selector/3 -> Data Type Conversion/1  "<HeadingAngle>"
  Bus Selector/4 -> Data Type Conversion1/1  "<LateralDeviation>"
  Data Type Conversion1/1 -> Unary Minus1/1
  Bus Selector/1 -> Data Type Conversion3/1  "<Curvature>"
  Bus Selector/2 -> Data Type Conversion2/1  "<CurvatureDerivative>"
  Longitudinal Velocity/1 -> Product/2
  Unary Minus/1 -> Saturation1/1
  Saturation/1 -> Lateral Deviation/1
  Saturation1/1 -> Relative Yaw Angle/1
  Saturation3/1 -> Product/1
  Product/1 -> Gain/1
  Sum/1 -> Previewed Curvature/1
  Gain/1 -> Sum/2
  Saturation2/1 -> Sum/1
  Data Type Conversion/1 -> Unary Minus/1
  Data Type Conversion2/1 -> Saturation3/1
  Data Type Conversion3/1 -> Saturation2/1
  CoordinateChange/1(LaneCenter_SAE) -> Bus Selector/1
  Unary Minus1/1 -> Saturation/1

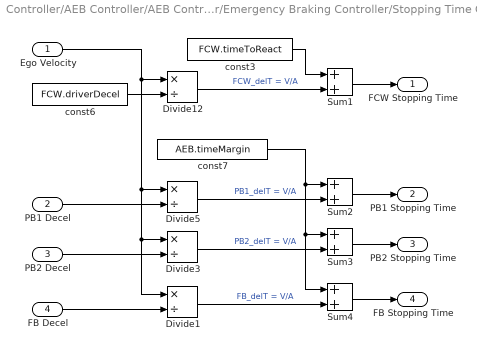
== system Controller/AEB Controller/AEB Controller/Emergency Braking Controller/Stopping Time Calculation ==
  Ego Velocity : Inport  SampleTime=ControllerStepSize
  PB1 Decel : Inport  Port=2
  PB2 Decel : Inport  Port=3
  FB Decel : Inport  Port=4
  Divide{1,3,5,12} (4 alike) : Product  Inputs=*/
  Sum{1..4} (4 alike) : Sum
  const3 : Constant  Value=FCW.timeToReact  SampleTime=-1
  const6 : Constant  Value=FCW.driverDecel  SampleTime=-1
  const7 : Constant  Value=AEB.timeMargin  SampleTime=-1
  FCW Stopping Time : Outport  VectorParamsAs1DForOutWhenUnconnected=off
  PB1 Stopping Time : Outport  Port=2  VectorParamsAs1DForOutWhenUnconnected=off
  PB2 Stopping Time : Outport  Port=3  VectorParamsAs1DForOutWhenUnconnected=off
  FB Stopping Time : Outport  Port=4  VectorParamsAs1DForOutWhenUnconnected=off
  wires:
  Sum1/1 -> FCW Stopping Time/1
  Sum2/1 -> PB1 Stopping Time/1
  Sum3/1 -> PB2 Stopping Time/1
  Sum4/1 -> FB Stopping Time/1
  const7/1 -> Sum2/1, Sum4/1, Sum3/1
  Ego Velocity/1 -> Divide1/1, Divide3/1, Divide5/1, Divide12/1
  Divide5/1 -> Sum2/2  "PB1_delT = V/A"
  Divide3/1 -> Sum3/2  "PB2_delT = V/A"
  Divide1/1 -> Sum4/2  "FB_delT = V/A"
  const6/1 -> Divide12/2
  PB1 Decel/1 -> Divide5/2
  PB2 Decel/1 -> Divide3/2
  FB Decel/1 -> Divide1/2
  const3/1 -> Sum1/1
  Divide12/1 -> Sum1/2  "FCW_delT = V/A"

== system Controller/AEB Controller/AEB Controller/Emergency Braking Controller/TTC Calculation ==
  Mio Distance : Inport
  Mio Velocity : Inport  Port=2
  Abs : Abs  SaturateOnIntegerOverflow=off
  Divide11 : Product  Inputs=**
  Divide3 : Product  Inputs=*/
  Saturation : Saturate  UpperLimit=100  LowerLimit=0.01
  Sign : Signum
  Sum : Sum  Inputs=+-
  const1 : Constant  Value=AEB.headwayOffset  SampleTime=-1
  TTC : Outport  VectorParamsAs1DForOutWhenUnconnected=off
  wires:
  Mio Velocity/1 -> Sign/1, Abs/1
  Mio Distance/1 -> Sum/1
  Divide3/1 -> Divide11/1  "TTC"
  const1/1 -> Sum/2
  Sum/1 -> Divide3/1  "headway"
  Abs/1 -> Saturation/1
  Saturation/1 -> Divide3/2
  Sign/1 -> Divide11/2
  Divide11/1 -> TTC/1

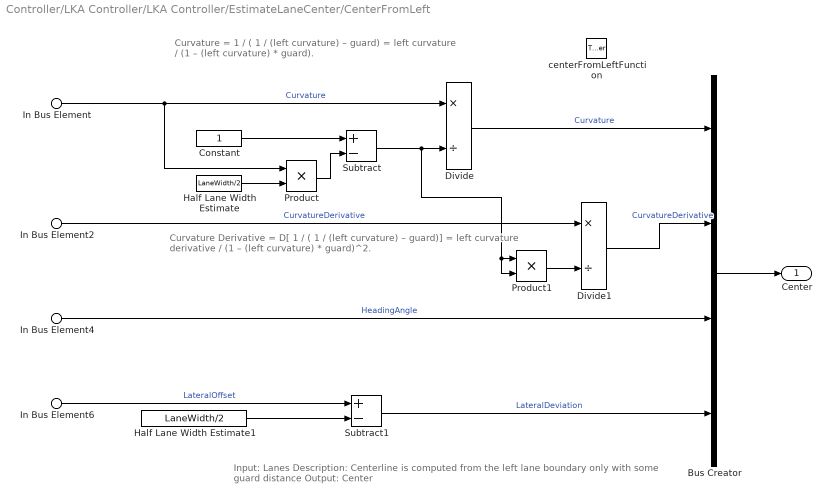
== system Controller/LKA Controller/LKA Controller/EstimateLaneCenter/CenterFromLeft ==
  note: Curvature Derivative
      | = D[ 1 / ( 1 / (left curvature) – guard)]
      | = left curvature derivative / (1 – (left curvature) * guard)^2.
  note: Curvature
      | = 1 / ( 1 / (left curvature) – guard)
      | = left curvature / (1 – (left curvature) * guard).
  note: Input: Lanes
      | Description: Centerline is computed from the left lane boundary only with some guard distance
      | Output: Center
  In Bus Element : Inport  PortName=Lanes  Element=Left.Curvature
  In Bus Element2 : Inport  PortName=Lanes  Element=Left.CurvatureDerivative
  In Bus Element4 : Inport  PortName=Lanes  Element=Left.HeadingAngle
  In Bus Element6 : Inport  PortName=Lanes  Element=Left.LateralOffset
  centerFromLeftFunction : TriggerPort  TriggerType=function-call  VariantControl=Variant
  Bus Creator : BusCreator  Inputs=4
  Constant : Constant  OutDataTypeStr=Inherit: Inherit via back propagation
  Divide : Product  Inputs=*/
  Divide1 : Product  Inputs=*/
  Half Lane Width Estimate : Constant  Value=LaneWidth/2  OutDataTypeStr=Inherit: Inherit via back propagation
  Half Lane Width Estimate1 : Constant  Value=LaneWidth/2  OutDataTypeStr=Inherit: Inherit via back propagation
  Product : Product
  Product1 : Product
  Subtract : Sum  Inputs=+-
  Subtract1 : Sum  Inputs=+-
  Center : Outport  VectorParamsAs1DForOutWhenUnconnected=off
  wires:
  Product/1 -> Subtract/2
  Half Lane Width Estimate1/1 -> Subtract1/2
  In Bus Element6/1 -> Subtract1/1  "LateralOffset"
  Product1/1 -> Divide1/2
  In Bus Element2/1 -> Divide1/1  "CurvatureDerivative"
  Constant/1 -> Subtract/1
  Half Lane Width Estimate/1 -> Product/2
  Subtract/1 -> Divide/2, Product1/1, Product1/2
  In Bus Element/1 -> Divide/1, Product/1  "Curvature"
  Subtract1/1 -> Bus Creator/4  "LateralDeviation"
  In Bus Element4/1 -> Bus Creator/3  "HeadingAngle"
  Divide/1 -> Bus Creator/1  "Curvature"
  Divide1/1 -> Bus Creator/2  "CurvatureDerivative"
  Bus Creator/1 -> Center/1

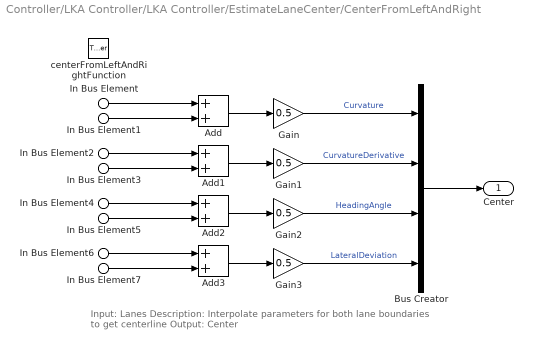
== system Controller/LKA Controller/LKA Controller/EstimateLaneCenter/CenterFromLeftAndRight ==
  note: Input: Lanes
      | Description: Interpolate parameters for both lane boundaries to get centerline
      | Output: Center
  In Bus Element : Inport  PortName=Lanes  Element=Left.Curvature
  In Bus Element2 : Inport  PortName=Lanes  Element=Left.CurvatureDerivative
  In Bus Element4 : Inport  PortName=Lanes  Element=Left.HeadingAngle
  In Bus Element6 : Inport  PortName=Lanes  Element=Left.LateralOffset
  In Bus Element1 : Inport  PortName=Lanes  Element=Right.Curvature
  In Bus Element3 : Inport  PortName=Lanes  Element=Right.CurvatureDerivative
  In Bus Element5 : Inport  PortName=Lanes  Element=Right.HeadingAngle
  In Bus Element7 : Inport  PortName=Lanes  Element=Right.LateralOffset
  centerFromLeftAndRightFunction : TriggerPort  TriggerType=function-call  VariantControl=Variant
  Add{,1..3} (4 alike) : Sum
  Bus Creator : BusCreator  Inputs=4
  Gain{,1..3} (4 alike) : Gain  Gain=0.5
  Center : Outport  VectorParamsAs1DForOutWhenUnconnected=off
  wires:
  In Bus Element6/1 -> Add3/1
  In Bus Element7/1 -> Add3/2
  In Bus Element5/1 -> Add2/2
  In Bus Element4/1 -> Add2/1
  In Bus Element3/1 -> Add1/2
  In Bus Element2/1 -> Add1/1
  In Bus Element1/1 -> Add/2
  In Bus Element/1 -> Add/1
  Bus Creator/1 -> Center/1
  Gain3/1 -> Bus Creator/4  "LateralDeviation"
  Add3/1 -> Gain3/1
  Gain2/1 -> Bus Creator/3  "HeadingAngle"
  Add2/1 -> Gain2/1
  Gain1/1 -> Bus Creator/2  "CurvatureDerivative"
  Add1/1 -> Gain1/1
  Gain/1 -> Bus Creator/1  "Curvature"
  Add/1 -> Gain/1

== system Controller/LKA Controller/LKA Controller/EstimateLaneCenter/CenterFromNone ==
  note: Input: Lanes
      | Description: If current lane detections are not reliable, consider previous centerline as current
      | Output: Center
  OldCenter : Inport
      settings: LatchInputForFeedbackSignals=on
  centerFromNoneFunction : TriggerPort  TriggerType=function-call  VariantControl=Variant
  Delay : Delay  DelayLength=1
  NewCenter : Outport  VectorParamsAs1DForOutWhenUnconnected=off
  wires:
  OldCenter/1 -> Delay/1
  Delay/1 -> NewCenter/1

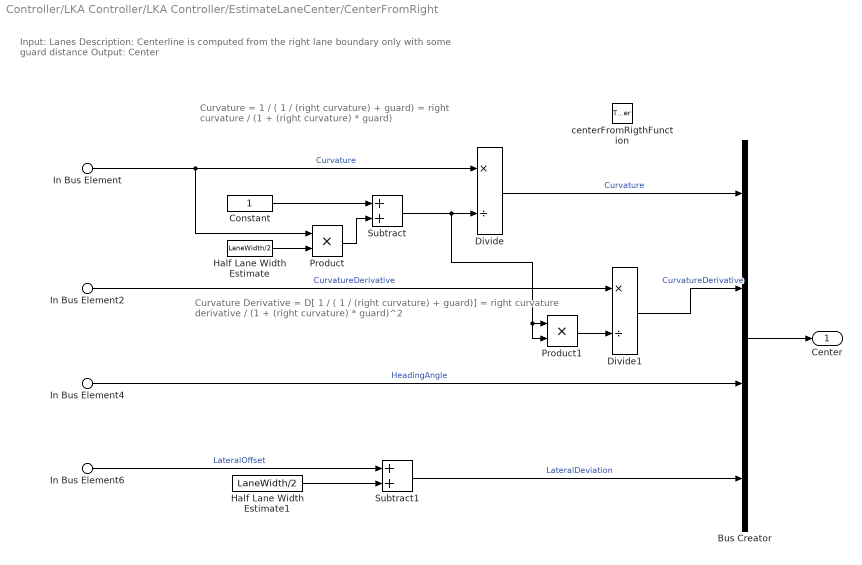
== system Controller/LKA Controller/LKA Controller/EstimateLaneCenter/CenterFromRight ==
  note: Curvature Derivative
      | = D[ 1 / ( 1 / (right curvature) + guard)]
      | = right curvature derivative / (1 + (right curvature) * guard)^2
  note: Curvature
      | = 1 / ( 1 / (right curvature) + guard)
      | = right curvature / (1 + (right curvature) * guard)
  note: Input: Lanes
      | Description: Centerline is computed from the right lane boundary only with some guard distance
      | Output: Center
  In Bus Element : Inport  PortName=Lanes  Element=Right.Curvature
  In Bus Element2 : Inport  PortName=Lanes  Element=Right.CurvatureDerivative
  In Bus Element4 : Inport  PortName=Lanes  Element=Right.HeadingAngle
  In Bus Element6 : Inport  PortName=Lanes  Element=Right.LateralOffset
  centerFromRigthFunction : TriggerPort  TriggerType=function-call  VariantControl=Variant
  Bus Creator : BusCreator  Inputs=4
  Constant : Constant  OutDataTypeStr=Inherit: Inherit via back propagation
  Divide : Product  Inputs=*/
  Divide1 : Product  Inputs=*/
  Half Lane Width Estimate : Constant  Value=LaneWidth/2  OutDataTypeStr=Inherit: Inherit via back propagation
  Half Lane Width Estimate1 : Constant  Value=LaneWidth/2  OutDataTypeStr=Inherit: Inherit via back propagation
  Product : Product
  Product1 : Product
  Subtract : Sum
  Subtract1 : Sum
  Center : Outport  VectorParamsAs1DForOutWhenUnconnected=off
  wires:
  Half Lane Width Estimate/1 -> Product/2
  Product/1 -> Subtract/2
  Constant/1 -> Subtract/1
  Subtract/1 -> Divide/2, Product1/1, Product1/2
  In Bus Element/1 -> Divide/1, Product/1  "Curvature"
  Bus Creator/1 -> Center/1
  Subtract1/1 -> Bus Creator/4  "LateralDeviation"
  Divide/1 -> Bus Creator/1  "Curvature"
  In Bus Element6/1 -> Subtract1/1  "LateralOffset"
  Half Lane Width Estimate1/1 -> Subtract1/2
  In Bus Element4/1 -> Bus Creator/3  "HeadingAngle"
  Product1/1 -> Divide1/2
  Divide1/1 -> Bus Creator/2  "CurvatureDerivative"
  In Bus Element2/1 -> Divide1/1  "CurvatureDerivative"

== system Controller/LKA Controller/LKA Controller/Preview Curvature/CoordinateChange ==
  note: Input: LaneCenter_ISO
      | Description: change lane center representation from the ISO 8855 to SAE J670E coordinate system. In ISO 8855 positive Y is to the left, whereas it is to the right in SAE J670E
      | Output: LaneCenter_SAE
  LaneCenter_ISO : Inport
  Bus Creator : BusCreator  Inputs=4
  Bus Selector : BusSelector  OutputSignals=CurvatureDerivative,Curvature,HeadingAngle,LateralDeviation
  Signal Specification : SignalSpecification  Unit=1/m^2
  Signal Specification1 : SignalSpecification  Unit=1/m
  Signal Specification2 : SignalSpecification  Unit=rad
  Signal Specification3 : SignalSpecification  Unit=m
  Unary Minus{,1..3} (4 alike) : UnaryMinus
  LaneCenter_SAE : Outport  VectorParamsAs1DForOutWhenUnconnected=off
  wires:
  Signal Specification3/1 -> Bus Creator/4  "LateralDeviation"
  Signal Specification2/1 -> Bus Creator/3  "HeadingAngle"
  Signal Specification/1 -> Bus Creator/1  "CurvatureDerivative"
  Unary Minus/1 -> Signal Specification1/1
  Unary Minus3/1 -> Signal Specification3/1
  Unary Minus2/1 -> Signal Specification2/1
  Unary Minus1/1 -> Signal Specification/1
  Signal Specification1/1 -> Bus Creator/2  "Curvature"
  Bus Creator/1 -> LaneCenter_SAE/1
  Bus Selector/4 -> Unary Minus3/1  "<LateralDeviation>"
  Bus Selector/3 -> Unary Minus2/1  "<HeadingAngle>"
  Bus Selector/1 -> Unary Minus1/1  "<CurvatureDerivative>"
  Bus Selector/2 -> Unary Minus/1  "<Curvature>"
  LaneCenter_ISO/1 -> Bus Selector/1

== matlab function Controller/AEB Controller/AEB Controller/Find MIO ==
  data: confirmedTracks input Bus: BusMultiObjectTracker1; x output size=[1 1]; vx output size=[1 1]; mioTrack output; positionSelector input; laneWidth input; relativeYawAngle output; egoSpeed input
function [x,vx,mioTrack, relativeYawAngle] = findMIO(confirmedTracks, positionSelector, laneWidth, egoSpeed)
% This function finds the lead car: a car in front of the ego car that
% satisfies all the criteria below:
% * Within the ego car's lane.
% * In front of the ego car.
% * Closest to the ego car.

% Important notes:
% 1. If you change state definition, change the following:
%       State = [x;vx;y;vy;z;vz] (3D constant velocity)
numStates = 6;
relativeYawAngle =0 ;
% 2. The ego car is assumed to be traveling in the middle of its lane.
halfLaneWidth = laneWidth/2;

% Initialize outputs and parameters
maxX = cast(1000, 'like', confirmedTracks.Tracks(1).State);  % Far enough forward so that no track is expected to exceed this distance
trackID = 0;
crossingTargetLateralDist = 18;
targetCollisionThresholdTime = 2; % Collision threshold time beyond which the target should be treated as MIO 
stationaryVelocityThreshold = eps('single'); % Threshold to determine if a target is effectively stationary relative to the world

for i = 1:confirmedTracks.NumTracks
    position = positionSelector * confirmedTracks.Tracks(i).State;
    x = position(1); % Longitudinal position of the track relative to ego
    y = position(2); % Lateral position of the track relative to ego

    if x < maxX && x > 0 % No point checking otherwise
        % Detect cross target as MIO to avoid collision
        
        if (-crossingTargetLateralDist <= y) && (y <= crossingTargetLateralDist) &&  ...
                abs(norm([confirmedTracks.Tracks(i).State(2), confirmedTracks.Tracks(i).State(4), confirmedTracks.Tracks(i).State(6)]) - egoSpeed) >= stationaryVelocityThreshold
            estimatedCollisionTime = confirmedTracks.Tracks(i).State(1)/abs(confirmedTracks.Tracks(i).State(2));
            if(targetCollisionThresholdTime>abs(estimatedCollisionTime))
                maxX = x;
                trackID = i;
            end
        end

        yleftLane  = polyval([0, 0,  halfLaneWidth],x); % Half a lane to the left
        yrightLane = polyval([0, 0, -halfLaneWidth],x); % Half a lane to the right
        % Find a new lead car
        if (yrightLane <= y) && (y <= yleftLane)
            maxX = x;
            trackID = i;
        end
    end
end

if trackID>0
    mioState = confirmedTracks.Tracks(trackID).State;
    relativeYawEgoFrame = atan2(mioState(4), mioState(2));
    relativeYawAngle = relativeYawEgoFrame;
else
    mioState = zeros(numStates,1,'like',confirmedTracks.Tracks(1).State);
    mioState(1) = 500;
    mioState(2) = 0.01;
end

% Output:
x = mioState(1);    % Longitudinal position of the lead car
vx = mioState(2);   % Longitudinal velocity of the lead car
mioTrack = trackID; % Index of the most important track

== stateflow chart Controller/AEB Controller/AEB Controller/Emergency Braking Controller/AEB Logic ==
  note: FCW/AEB Logic
  state Default
    entry: AEBstatus = 0;
    FCWactivate = 0;
    decel = 0;
  state FCW
    entry: AEBstatus = 0;
    FCWactivate = 1;
    decel = 0;
  state Partial_Braking1
    entry: AEBstatus = 1;
    FCWactivate = 1;
    decel = PB1decel;
  state Full_Braking
    entry: AEBstatus = 3;
    FCWactivate = 1;
    decel = FBdecel;
  state Partial_Braking2
    entry: AEBstatus = 2;
    FCWactivate = 1;
    decel = PB2decel;
  (default) -> Default
  (junction 78) -> Default
  Full_Braking -> (junction 78) [order 1] : [stop==1]
  (junction 80) -> Default
  (junction 90) -> (junction 80) : [stop==1]
  (junction 86) -> Default
  (junction 88) -> (junction 86)
  Default -> FCW : [(abs(TTC)<FCWtime) && TTC<0.6&&stop~=1]
  FCW -> (junction 76) [order 1]
  (junction 76) -> Full_Braking : [ abs(relativeYawAngle) >= deg2rad(89) && TTC<0.6 && ...
      | Mio_Distance < defaultSpacing && ...
      | stop~=1]
  FCW -> Partial_Braking1 [order 2] : [(abs(TTC) < PB1time) && TTC<0&&stop~=1]
  Partial_Braking1 -> (junction 88) [order 2] : [stop==1]
  Partial_Braking1 -> Partial_Braking2 [order 1] : [(abs(TTC) < PB2time) && TTC<0&&stop~=1]
  Partial_Braking2 -> Partial_Braking1 [order 2] : [abs(TTC)>=1.2*PB2time]
  Partial_Braking2 -> (junction 90) [order 1]
  Full_Braking -> Partial_Braking2 [order 2] : [abs(TTC)>=3*FBtime]
  Partial_Braking2 -> Full_Braking [order 3] : [(abs(TTC) < FBtime) && TTC<0&&stop~=1]
  data: FCWactivate output uint8; TTC input; FCWtime input; PB1time input; PB2time input; FBtime input; PB1decel input; PB2decel input; FBdecel input; AEBstatus output uint8; decel output; stop input; Mio_Distance input; defaultSpacing parameter; relativeYawAngle input

== matlab function Controller/LKA Controller/LKA Controller/Ego Speed ==
  data: speed output; velocity input
function speed = egoSpeed(velocity)

speed = norm([velocity(1), velocity(2), velocity(3)]);

== matlab function Controller/LKA Controller/LKA Controller/EstimateLaneCenter/MATLAB Function ==
  data: lanes input
  events: centerFromLeftAndRightFunction output FUNCTION_CALL_EVENT; centerFromLeftFunction output FUNCTION_CALL_EVENT; centerFromRigthFunction output FUNCTION_CALL_EVENT; centerFromNoneFunction output FUNCTION_CALL_EVENT
function fcn(lanes)

leftStrength  = lanes.Left.Strength;
rightStrength = lanes.Right.Strength;

if (leftStrength > 0) && (rightStrength > 0)
   centerFromLeftAndRightFunction();
   
elseif leftStrength > 0
    centerFromLeftFunction();
    
elseif rightStrength > 0
    centerFromRigthFunction();
    
else
    centerFromNoneFunction();
end

== matlab function Controller/AEB Controller/AEB Controller/Ego Speed ==
  data: speed output; velocity input
function speed = egoSpeed(velocity)

speed = norm([velocity(1), velocity(2), velocity(3)]);

== matlab function Controller/LKA Controller/LKA Controller/Pack Lane Detections/MATLAB Function ==
  data: laterOffset input; strengthOut output; strength input
function strengthOut = fcn(laterOffset,strength)

if isnan(laterOffset)
    strengthOut = 0;
else
    strengthOut = strength;
end

== matlab function Controller/LKA Controller/LKA Controller/Pack Lane Detections/MATLAB Function1 ==
  data: laterOffset input; strengthOut output; strength input
function strengthOut = fcn(laterOffset,strength)

if isnan(laterOffset)
    strengthOut = 0;
else
    strengthOut = strength;
end

== matlab function Controller/Trajectory Following Controller/MATLAB Function ==
  data: currentPose output; pose input; speed output
function [currentPose, speed] = egoPose(pose)

speed = hypot(pose.Velocity(1),pose.Velocity(2));
currentPose = [pose.Position(1), pose.Position(2), pose.Yaw];
end

== matlab function Controller/ACC Longitudinal Controller/Select Lead Vehicle ==
  data: tracks input Bus: BusMultiObjectTracker1 size=1; distance output size=1; egoVelocity input size=[1 3]; laneWidth input size=1; relativeSpeed output size=1; egoSpeed output size=1
function [distance, relativeSpeed, egoSpeed] = selectLead(tracks, egoVelocity, laneWidth)
% Select the closest tracked vehicle ahead in the ego lane.
egoSpeed = hypot(egoVelocity(1), egoVelocity(2));
distance = 500;
relativeSpeed = 0;
halfLaneWidth = laneWidth/2;
for idx = 1:20
    if idx <= tracks.NumTracks
        state = tracks.Tracks(idx).State;
        longitudinalDistance = state(1);
        lateralDistance = state(3);
        if longitudinalDistance > 0 && longitudinalDistance < distance && abs(lateralDistance) <= halfLaneWidth
            distance = longitudinalDistance;
            relativeSpeed = state(2);
        end
    end
end
end
